simulink model "cbuildv3p1"  (R2024b)
settings: Solver=VariableStepAuto  StartTime=0.0  StopTime=2  RelTol=1e-3
model workspace (MAT data in the model file):
  A_busbar = 0.0015
  A_pack = 0.711626248
  C = 400
  C_nominal = 3
  GR = 13.75
  I_max = 157.708978328
  Izz = 76.97
  M = 251.54
  P = 5
  P_DD = 1
  REGEN_GAIN = 1
  R_e = 0.195
  S = 138
  SW_TV_GAIN = 0.0250298750679
  SoC_initial = 1
  TC_CUT = 500
  T_amb = 297.15
  Tmax = 21
  W = 1.53
  W_max = 34
  a = 0.7497
  busbar_CC_area = 0.000108
  busbar_Cp = 237
  busbar_length = 0.032
  busbar_mass = 0.01
  busbar_resistivity = 1.68e-08
  busbar_thermalcontact_resistance = 1
  c_factor = 0.244
  cell_Cp = 1000
  cell_mass = 0.046
  deg_to_rad = 0.0174533
  g = 9.81
  h = 0.253
  h_busbar = 5
  h_pack = 5
  kappa_thresh = 0.05
  l = 1.53
  mpersec_to_kph = 3.6
  rackdisp_to_steerangle = 1.29615626969
  rad_to_deg = 57.2958
  rpm_to_radpers = 0.10472
  t = 1.2
libraries: Solver_SF x1
(part 1 of 2)
settings Model: Creator=account  LastModifiedBy=kara.28

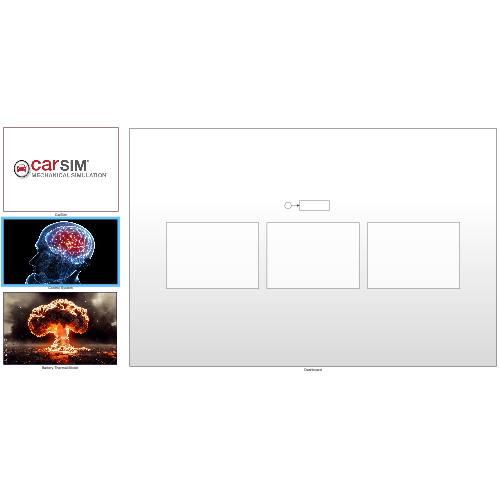
[thumbnail: Simulink's stored preview of the top-level diagram]
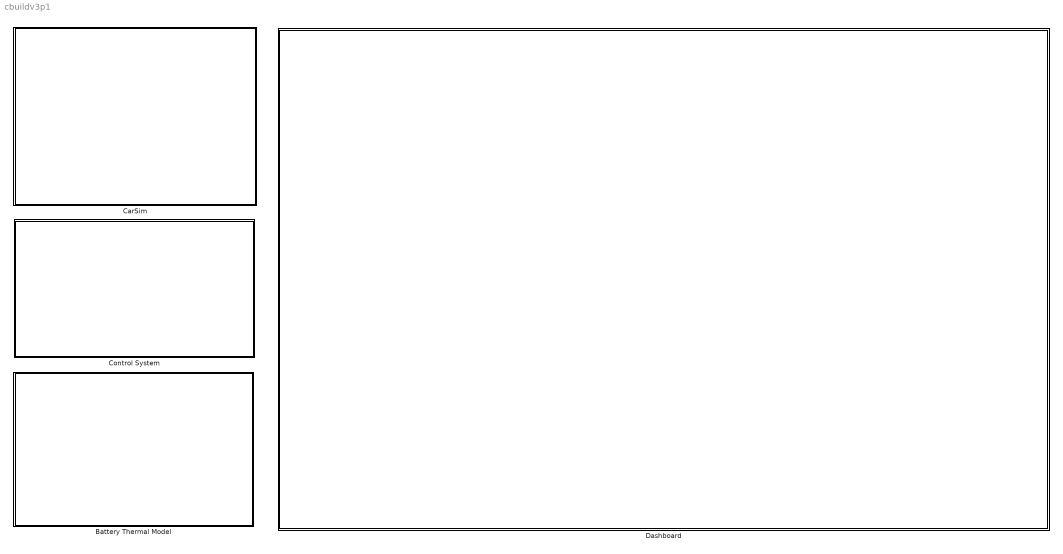
== system cbuildv3p1 ==
  Battery Thermal Model : Subsystem
      mask Display: image('battery.jpg');
  CarSim : Subsystem
      mask Display: image('carsimlogo.jpg');
  Control System : Subsystem
      mask Display: image('controller.jpg');
  Dashboard : Subsystem

== system cbuildv3p1/Battery Thermal Model ==
  Battery Cells : Subsystem
  Busbars : Subsystem

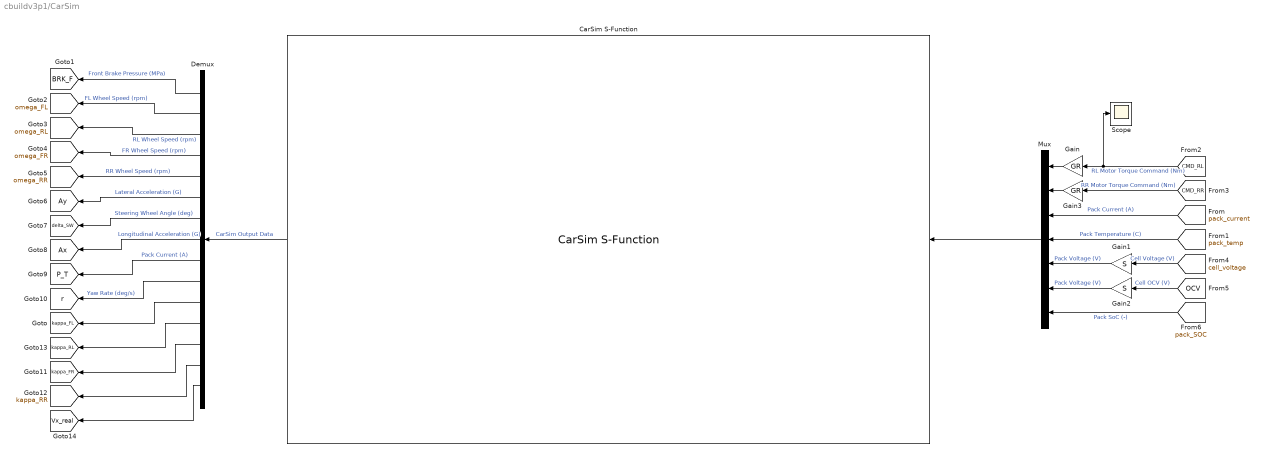
== system cbuildv3p1/CarSim ==
  CarSim S-Function : Solver_SF/CarSim S-Function  Priority=1  SIMFILE=simfile.sim  Run_RTs=off  vs_state_ind=Run  StopMode_ind=Vehicle Model
  Demux : Demux  Outputs=15
  Gain : Gain  Gain=GR
  Gain1 : Gain  Gain=S
  Gain2 : Gain  Gain=S
  Gain3 : Gain  Gain=GR
  Mux : Mux  Inputs=7
  Scope : Scope
  tag scope: Ax=global, Ay=global, BRK_F=global, P_T=global, Vx_real=global, delta_SW=global, kappa_FL=global, kappa_FR=global, kappa_RL=global, kappa_RR=global, omega_FL=global, omega_FR=global, omega_RL=global, omega_RR=global, r=global
  wires:
  Demux/5 -> [omega_RR]  "RR Wheel Speed (rpm)"
  Demux/8 -> [Ax]  "Longitudinal Acceleration (G)"
  Demux/4 -> [omega_FR]  "FR Wheel Speed (rpm)"
  Demux/2 -> [omega_FL]  "FL Wheel Speed (rpm)"
  CarSim S-Function/1 -> Demux/1  "CarSim Output Data"
  Demux/7 -> [delta_SW]  "Steering Wheel Angle (deg)"
  [CMD_RR] -> Gain3/1  "RR Motor Torque Command (Nm)"
  [CMD_RL] -> Scope/1, Gain/1  "RL Motor Torque Command (Nm)"
  Demux/3 -> [omega_RL]  "RL Wheel Speed (rpm)"
  Demux/1 -> [BRK_F]  "Front Brake Pressure (MPa)"
  Demux/6 -> [Ay]  "Lateral Acceleration (G)"
  Mux/1 -> CarSim S-Function/1
  Demux/10 -> [r]  "Yaw Rate (deg/s)"
  [pack_current] -> Mux/3  "Pack Current (A)"
  [pack_temp] -> Mux/4  "Pack Temperature (C)"
  [pack_SOC] -> Mux/7  "Pack SoC (-)"
  [OCV] -> Gain2/1  "Cell OCV (V)"
  [cell_voltage] -> Gain1/1  "Cell Voltage (V)"
  Gain1/1 -> Mux/5  "Pack Voltage (V)"
  Gain2/1 -> Mux/6  "Pack Voltage (V)"
  Gain/1 -> Mux/1
  Gain3/1 -> Mux/2
  Demux/9 -> [P_T]  "Pack Current (A)"
  Demux/11 -> [kappa_FL]
  Demux/12 -> [kappa_RL]
  Demux/13 -> [kappa_FR]
  Demux/14 -> [kappa_RR]
  Demux/15 -> [Vx_real]

== system cbuildv3p1/Control System ==
  Driver Assists : Subsystem
      settings: PortSchema="{\"entries\":[{\"content\":{\"sides\":[{\"content\":{\"connectorIds\":[\"In1\",\"In2\"]},\"type\":\"ConnectorPlacement.EquallySpacedRectSide\",\"uuid\":\"c30f5bbb-5f7b-4b8f-a220-579b9cc0865f\"},{\"content\":{\"connectorIds\":[\"Out1\",\"Out2\"],\"side\":\"RIGHT\"},\"type\":\"ConnectorPlacement.EquallySpacedRectSide\",\"uuid\":\"8399a92e-19c3-49c4-801c-f7e7f76799cf\"},{\"content\":{\"connectorIds\":[\"In3\",\"In4\",\"In5\",\"In6\",\"In7\",\"In8\",\"In9\"],\"side\":\"TOP\"},\"type\":\"ConnectorPlacement.EquallySpacedRectSide\",\"uuid\":\"19d8375b-8353-4f23-adee-fcd0b0fbd4ef\"}]},\"type\":\"ConnectorPlacement.EquallySpacedConnector\",\"uuid\":\"53834b5a-6686-42bc-a078-9cae71bfd001\"}],\"packageUris\":[\"http://schema.mathworks.com/mf0/Connector/R2020b\"],\"version\":\"1.0\"}"
  Dynamic Derate Dial Position : Constant
  Energy Management System : Subsystem
      settings: PortSchema="{\"entries\":[{\"content\":{\"sides\":[{\"content\":{\"connectorIds\":[\"In1\",\"In2\"]},\"type\":\"ConnectorPlacement.EquallySpacedRectSide\",\"uuid\":\"89c92abe-ca77-4c48-ba79-1fd8447b36ee\"},{\"content\":{\"connectorIds\":[\"Out1\",\"Out2\"],\"side\":\"RIGHT\"},\"type\":\"ConnectorPlacement.EquallySpacedRectSide\",\"uuid\":\"4a58accb-bbe3-490f-b1ea-5257f75ab2ba\"},{\"content\":{\"connectorIds\":[\"In3\",\"In4\",\"In5\"],\"side\":\"TOP\"},\"type\":\"ConnectorPlacement.EquallySpacedRectSide\",\"uuid\":\"b5e96e52-1098-4ccd-9740-b2b10d8cf6b3\"}]},\"type\":\"ConnectorPlacement.EquallySpacedConnector\",\"uuid\":\"06c6d35a-fc7b-4382-b862-8bbe65743431\"}],\"packageUris\":[\"http://schema.mathworks.com/mf0/Connector/R2020b\"],\"version\":\"1.0\"}"
  tag scope: CMD_RL=global, CMD_RR=global
  wires:
  Energy Management System/1(CMD_R) -> Driver Assists/1(CMD_R)
  Energy Management System/2(Tmax) -> Driver Assists/2(Tmax)
  Driver Assists/1(CMD_RL) -> [CMD_RL]
  Driver Assists/2(CMD_RR) -> [CMD_RR]
  [pack_temp] -> Energy Management System/1(T_BAT_MAX)  "Battery Temp (C)"
  Dynamic Derate Dial Position/1 -> Energy Management System/2(P_DD)  "Derate Dial Position (-)"
  [omega_RR] -> Driver Assists/6(omega_RR), Energy Management System/5(omega_RR)  "RR Wheel Speed (rpm)"
  [omega_FR] -> Driver Assists/4(omega_FR)  "FR Wheel Speed (rpm)"
  [omega_RL] -> Driver Assists/5(omega_RL), Energy Management System/3(omega_RL)  "RL Wheel Speed (rpm)"
  [omega_FL] -> Driver Assists/3(omega_FL)  "FL Wheel Speed (rpm)"
  [P_T] -> Driver Assists/7(P_T)  "Throttle Position (-)"
  [Ay] -> Driver Assists/8(Ax)  "Lateral Acceleration (G)"
  [BRK_F] -> Energy Management System/4(BRK_F), Driver Assists/9(BRK_F)  "Front Brake Pressure (MPa)"

== system cbuildv3p1/Dashboard ==
  Battery Info : Subsystem
  Clock1 : Clock
  Controls Info : Subsystem
  General Info : Subsystem
  Simulation Time : Display
  wires:
  Clock1/1 -> Simulation Time/1

== system cbuildv3p1/Battery Thermal Model/Battery Cells ==
  Battery Heat : Subsystem
      settings: PortSchema="{\"entries\":[{\"content\":{\"sides\":[{\"content\":{\"connectorIds\":[\"In1\",\"Out1\",\"In2\",\"In3\"]},\"type\":\"ConnectorPlacement.EquallySpacedRectSide\",\"uuid\":\"0f7c0562-63f7-413a-9c65-7d5d0f23ac53\"},{\"content\":{\"side\":\"RIGHT\"},\"type\":\"ConnectorPlacement.EquallySpacedRectSide\",\"uuid\":\"6856fc4a-e601-47fb-aafe-3183d6398fa2\"},{\"content\":{\"side\":\"TOP\"},\"type\":\"ConnectorPlacement.EquallySpacedRectSide\",\"uuid\":\"93500152-ab0c-4e86-a765-8796b82b9cd6\"}]},\"type\":\"ConnectorPlacement.EquallySpacedConnector\",\"uuid\":\"8bef09a8-0835-4033-ba4e-3f5f6277d0ac\"}],\"packageUris\":[\"http://schema.mathworks.com/mf0/Connector/R2020b\"],\"version\":\"1.0\"}"
  Battery Heat Generation : Subsystem
  Busbar - Segment Heat Flow : Subsystem
      settings: PortSchema="{\"entries\":[{\"content\":{\"sides\":[{\"content\":{},\"type\":\"ConnectorPlacement.EquallySpacedRectSide\",\"uuid\":\"839c7b7c-3d90-4543-803d-828e2cd8ee3e\"},{\"content\":{\"connectorIds\":[\"In1\",\"Out1\"],\"side\":\"RIGHT\"},\"type\":\"ConnectorPlacement.EquallySpacedRectSide\",\"uuid\":\"e3492608-3f40-473c-8392-0c925b682872\"},{\"content\":{\"side\":\"TOP\"},\"type\":\"ConnectorPlacement.EquallySpacedRectSide\",\"uuid\":\"8e15337c-e61d-491c-b508-620217c9bb60\"}]},\"type\":\"ConnectorPlacement.EquallySpacedConnector\",\"uuid\":\"03d3ec16-7a24-4203-9805-446eb586226e\"}],\"packageUris\":[\"http://schema.mathworks.com/mf0/Connector/R2020b\"],\"version\":\"1.0\"}"
  Heat Loss : Subsystem
      settings: PortSchema="{\"entries\":[{\"content\":{\"sides\":[{\"content\":{},\"type\":\"ConnectorPlacement.EquallySpacedRectSide\",\"uuid\":\"cd11f8f0-ebc0-4dda-8c98-00f5919de41a\"},{\"content\":{\"connectorIds\":[\"In1\",\"Out1\"],\"side\":\"RIGHT\"},\"type\":\"ConnectorPlacement.EquallySpacedRectSide\",\"uuid\":\"2a68a9a1-bd97-4a17-8a8b-1aa98e9bd9a8\"},{\"content\":{\"side\":\"TOP\"},\"type\":\"ConnectorPlacement.EquallySpacedRectSide\",\"uuid\":\"debcc510-941b-4448-a371-f67c84c59f32\"}]},\"type\":\"ConnectorPlacement.EquallySpacedConnector\",\"uuid\":\"91559e46-754b-48b4-ac3e-ab135f9add0a\"}],\"packageUris\":[\"http://schema.mathworks.com/mf0/Connector/R2020b\"],\"version\":\"1.0\"}"
  wires:
  Battery Heat/1(Pack Temp (K)) -> Busbar - Segment Heat Flow/1(Segment Temp (K)), Heat Loss/1(Pack Temp (K))
  Battery Heat Generation/1(Battery Heat Generation Rate) -> Battery Heat/1(Battery Heat Generation)
  Heat Loss/1(Pack Heat Loss Rate) -> Battery Heat/2(Battery Heat Loss)
  Busbar - Segment Heat Flow/1(Busbar - Segment Heat Flow (W)) -> Battery Heat/3(Busbar - Segment Heat Flow (W))

== system cbuildv3p1/Battery Thermal Model/Busbars ==
  Ambient Heat Loss : Subsystem
      settings: PortSchema="{\"entries\":[{\"content\":{\"sides\":[{\"content\":{},\"type\":\"ConnectorPlacement.EquallySpacedRectSide\",\"uuid\":\"cd11f8f0-ebc0-4dda-8c98-00f5919de41a\"},{\"content\":{\"connectorIds\":[\"In1\",\"Out1\"],\"side\":\"RIGHT\"},\"type\":\"ConnectorPlacement.EquallySpacedRectSide\",\"uuid\":\"2a68a9a1-bd97-4a17-8a8b-1aa98e9bd9a8\"},{\"content\":{\"side\":\"TOP\"},\"type\":\"ConnectorPlacement.EquallySpacedRectSide\",\"uuid\":\"debcc510-941b-4448-a371-f67c84c59f32\"}]},\"type\":\"ConnectorPlacement.EquallySpacedConnector\",\"uuid\":\"91559e46-754b-48b4-ac3e-ab135f9add0a\"}],\"packageUris\":[\"http://schema.mathworks.com/mf0/Connector/R2020b\"],\"version\":\"1.0\"}"
  Busbar - Segment Heat Flow : Subsystem
      settings: PortSchema="{\"entries\":[{\"content\":{\"sides\":[{\"content\":{},\"type\":\"ConnectorPlacement.EquallySpacedRectSide\",\"uuid\":\"839c7b7c-3d90-4543-803d-828e2cd8ee3e\"},{\"content\":{\"connectorIds\":[\"In1\",\"Out1\"],\"side\":\"RIGHT\"},\"type\":\"ConnectorPlacement.EquallySpacedRectSide\",\"uuid\":\"e3492608-3f40-473c-8392-0c925b682872\"},{\"content\":{\"side\":\"TOP\"},\"type\":\"ConnectorPlacement.EquallySpacedRectSide\",\"uuid\":\"8e15337c-e61d-491c-b508-620217c9bb60\"}]},\"type\":\"ConnectorPlacement.EquallySpacedConnector\",\"uuid\":\"03d3ec16-7a24-4203-9805-446eb586226e\"}],\"packageUris\":[\"http://schema.mathworks.com/mf0/Connector/R2020b\"],\"version\":\"1.0\"}"
  Busbar Heat : Subsystem
      settings: PortSchema="{\"entries\":[{\"content\":{\"sides\":[{\"content\":{\"connectorIds\":[\"In1\",\"Out1\",\"In2\",\"In3\"]},\"type\":\"ConnectorPlacement.EquallySpacedRectSide\",\"uuid\":\"0f7c0562-63f7-413a-9c65-7d5d0f23ac53\"},{\"content\":{\"side\":\"RIGHT\"},\"type\":\"ConnectorPlacement.EquallySpacedRectSide\",\"uuid\":\"6856fc4a-e601-47fb-aafe-3183d6398fa2\"},{\"content\":{\"side\":\"TOP\"},\"type\":\"ConnectorPlacement.EquallySpacedRectSide\",\"uuid\":\"93500152-ab0c-4e86-a765-8796b82b9cd6\"}]},\"type\":\"ConnectorPlacement.EquallySpacedConnector\",\"uuid\":\"8bef09a8-0835-4033-ba4e-3f5f6277d0ac\"}],\"packageUris\":[\"http://schema.mathworks.com/mf0/Connector/R2020b\"],\"version\":\"1.0\"}"
  Resistance Heat Generation : Subsystem
  wires:
  Busbar Heat/1(Busbar Temp (K)) -> Busbar - Segment Heat Flow/1(Busbar Temp (K)), Ambient Heat Loss/1(Busbar Temp (K))
  Resistance Heat Generation/1(Busbar Heat Generation Rate) -> Busbar Heat/1(Busbar Heat Generation)
  Ambient Heat Loss/1(Busbar Heat Loss Rate) -> Busbar Heat/2(Busbar Heat Loss)
  Busbar - Segment Heat Flow/1(Busbar - Segment Heat Flow (W)) -> Busbar Heat/3(Busbar - Segment Heat Flow (W))

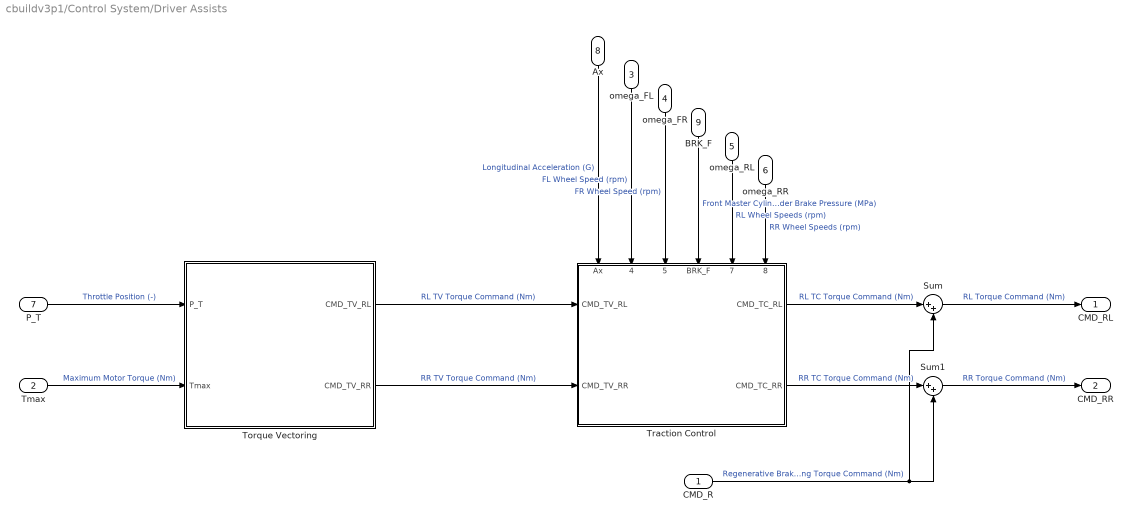
== system cbuildv3p1/Control System/Driver Assists ==
  CMD_R : Inport
  Tmax : Inport  Port=2
  omega_FL : Inport  Port=3
  omega_FR : Inport  Port=4
  omega_RL : Inport  Port=5
  omega_RR : Inport  Port=6
  P_T : Inport  Port=7
  Ax : Inport  Port=8
  BRK_F : Inport  Port=9
  Sum : Sum  Inputs=|++
  Sum1 : Sum  Inputs=|++
  Torque Vectoring : Subsystem
  Traction Control : Subsystem
      settings: PortSchema="{\"entries\":[{\"content\":{\"sides\":[{\"content\":{\"connectorIds\":[\"In1\",\"In2\"]},\"type\":\"ConnectorPlacement.EquallySpacedRectSide\",\"uuid\":\"d61c18bd-9535-4dda-869d-17effaf93de7\"},{\"content\":{\"connectorIds\":[\"Out1\",\"Out2\"],\"side\":\"RIGHT\"},\"type\":\"ConnectorPlacement.EquallySpacedRectSide\",\"uuid\":\"01ce504d-a060-4358-8411-664eedaba102\"},{\"content\":{\"connectorIds\":[\"In3\",\"In4\",\"In5\",\"In6\",\"In7\",\"In8\"],\"side\":\"TOP\"},\"type\":\"ConnectorPlacement.EquallySpacedRectSide\",\"uuid\":\"26eb6c05-86e8-47d0-a1b5-f53131bb5e60\"}]},\"type\":\"ConnectorPlacement.EquallySpacedConnector\",\"uuid\":\"a0cd41b8-03b3-4f62-a25e-73ac641935b2\"}],\"packageUris\":[\"http://schema.mathworks.com/mf0/Connector/R2020b\"],\"version\":\"1.0\"}"
  CMD_RL : Outport
  CMD_RR : Outport  Port=2
  wires:
  Torque Vectoring/2(CMD_TV_RR) -> Traction Control/2(CMD_TV_RR)  "RR TV Torque Command (Nm)"
  P_T/1 -> Torque Vectoring/1(P_T)  "Throttle Position (-)"
  Tmax/1 -> Torque Vectoring/2(Tmax)  "Maximum Motor Torque (Nm)"
  Sum/1 -> CMD_RL/1  "RL Torque Command (Nm)"
  Sum1/1 -> CMD_RR/1  "RR Torque Command (Nm)"
  CMD_R/1 -> Sum/2, Sum1/2  "Regenerative Braking Torque Command (Nm)"
  Ax/1 -> Traction Control/3(Ax)  "Longitudinal Acceleration (G)"
  omega_FL/1 -> Traction Control/4(omega_FL)  "FL Wheel Speed (rpm)"
  omega_FR/1 -> Traction Control/5(omega_FR)  "FR Wheel Speed (rpm)"
  BRK_F/1 -> Traction Control/6(BRK_F)  "Front Master Cylinder Brake Pressure (MPa)"
  omega_RL/1 -> Traction Control/7(omega_RL)  "RL Wheel Speeds (rpm)"
  omega_RR/1 -> Traction Control/8(omega_RR)  "RR Wheel Speeds (rpm)"
  Torque Vectoring/1(CMD_TV_RL) -> Traction Control/1(CMD_TV_RL)  "RL TV Torque Command (Nm)"
  Traction Control/1(CMD_TC_RL) -> Sum/1  "RL TC Torque Command (Nm)"
  Traction Control/2(CMD_TC_RR) -> Sum1/1  "RR TC Torque Command (Nm)"

== system cbuildv3p1/Control System/Energy Management System ==
  T_BAT_MAX : Inport
  P_DD : Inport  Port=2
  omega_RL : Inport  Port=3
  BRK_F : Inport  Port=4
  omega_RR : Inport  Port=5
  Dynamic Derate : Subsystem
  Regenerative Braking : Subsystem
  CMD_R : Outport
  Tmax : Outport  Port=2
  wires:
  T_BAT_MAX/1 -> Dynamic Derate/1(T_BAT_MAX)  "Maximum Module Temp (C)"
  P_DD/1 -> Dynamic Derate/2(P_DD)  "Dynamic Derate Dial Position (-)"
  BRK_F/1 -> Regenerative Braking/1(BRK_F)  "Front Master Cylinder Pressure (MPa)"
  Dynamic Derate/1(Tmax) -> Tmax/1  "Maximum Motor Torque (Nm)"
  Regenerative Braking/1(CMD_R) -> CMD_R/1  "Regen Brake Torque Command (Nm)"
  omega_RL/1 -> Dynamic Derate/3(omega_RL)  "RL Wheel Speed (rpm)"
  omega_RR/1 -> Dynamic Derate/4(omega_RR)  "RR Wheel Speed (rpm)"

== system cbuildv3p1/Dashboard/Battery Info ==
  Acceleration Scope : DashboardScope  Ymin=-2.5  Ymax=2.5
  Acceleration Scope1 : DashboardScope  Ymin=0  Ymax=60
  Acceleration Scope2 : DashboardScope  Ymin=0  Ymax=1
  Acceleration Scope3 : DashboardScope  Ymin=0  Ymax=1
  Acceleration Scope4 : DashboardScope  Ymin=0  Ymax=500

== system cbuildv3p1/Dashboard/Controls Info ==
  Acceleration Scope : DashboardScope  Ymin=-2.5  Ymax=2.5
  Acceleration Scope1 : DashboardScope  Ymin=-2  Ymax=2
  Acceleration Scope2 : DashboardScope  Ymin=0  Ymax=1
  Acceleration Scope3 : DashboardScope  Ymin=0  Ymax=80
  Acceleration Scope4 : DashboardScope  Ymin=0  Ymax=21
  Lamp : LampBlock  LabelPosition=Hide
  Rotary Switch : RotarySwitchBlock
      settings: Values={{'DD 1', 'DD 2'}, [0 1]}

== system cbuildv3p1/Dashboard/General Info ==
  Acceleration Scope : DashboardScope  Ymin=-2.5  Ymax=2.5
  Acceleration Scope1 : DashboardScope  Ymin=0  Ymax=110
  Acceleration Scope2 : DashboardScope  Ymin=0  Ymax=1
  Acceleration Scope3 : DashboardScope  Ymin=0  Ymax=10

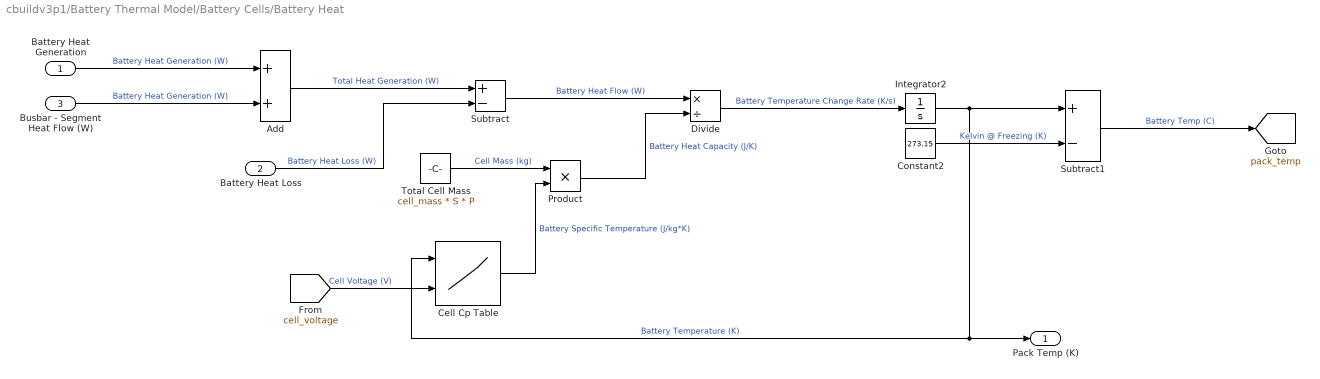
== system cbuildv3p1/Battery Thermal Model/Battery Cells/Battery Heat ==
  Battery Heat Generation : Inport
  Battery Heat Loss : Inport  Port=2
  Busbar - Segment Heat Flow (W) : Inport  Port=3
  Add : Sum
  Cell Cp Table : Lookup_n-D  BreakpointsForDimension1=[296.0488;303.3425;312.147;321.5769;330.6423]  BreakpointsForDimension2=[0 0.5 1]  Table=[811.0868 819.6535 830.8545;814.1373 822.704 834.6964;817.9826 826.8129 838.6737000000001;822.2249 831.0552 843.4446;826.7299 835.8239 848.3459]  InterpMethod=Cubic spline  InternalRulePriority=Speed  RndMeth=Simplest
      settings: InputPortMap=u0,u1
  Constant2 : Constant  Value=273.15
  Divide : Product  Inputs=*/
  Integrator2 : Integrator  InitialCondition=T_amb
  Product : Product
  Subtract : Sum  Inputs=+-
  Subtract1 : Sum  Inputs=+-
  Total Cell Mass : Constant  Value=cell_mass * S * P
  Pack Temp (K) : Outport
  tag scope: pack_temp=global
  wires:
  Cell Cp Table/1 -> Product/2  "Battery Specific Temperature (J/kg*K)"
  Constant2/1 -> Subtract1/2  "Kelvin @ Freezing (K)"
  Divide/1 -> Integrator2/1  "Battery Temperature Change Rate (K/s)"
  Subtract/1 -> Divide/1  "Battery Heat Flow (W)"
  Integrator2/1 -> Cell Cp Table/1, Pack Temp (K)/1, Subtract1/1  "Battery Temperature (K)"
  Subtract1/1 -> [pack_temp]  "Battery Temp (C)"
  Total Cell Mass/1 -> Product/1  "Cell Mass (kg)"
  Product/1 -> Divide/2  "Battery Heat Capacity (J/K)"
  Battery Heat Loss/1 -> Subtract/2  "Battery Heat Loss (W)"
  Battery Heat Generation/1 -> Add/1  "Battery Heat Generation (W)"
  Busbar - Segment Heat Flow (W)/1 -> Add/2  "Battery Heat Generation (W)"
  Add/1 -> Subtract/1  "Total Heat Generation (W)"
  [cell_voltage] -> Cell Cp Table/2  "Cell Voltage (V)"

== system cbuildv3p1/Battery Thermal Model/Battery Cells/Battery Heat Generation ==
  Cell Resistance : Subsystem
      settings: PortSchema="{\"entries\":[{\"content\":{\"sides\":[{\"content\":{},\"type\":\"ConnectorPlacement.EquallySpacedRectSide\",\"uuid\":\"1c6ff2a8-2c86-4b92-aa7d-5717a02d6f28\"},{\"content\":{\"connectorIds\":[\"In1\",\"In2\",\"Out1\"],\"side\":\"RIGHT\"},\"type\":\"ConnectorPlacement.EquallySpacedRectSide\",\"uuid\":\"52a4cb2c-e1db-459d-bd0a-206cc3bba6d1\"},{\"content\":{\"side\":\"TOP\"},\"type\":\"ConnectorPlacement.EquallySpacedRectSide\",\"uuid\":\"751bbbd6-abc7-4265-8d68-4aa70d69379f\"}]},\"type\":\"ConnectorPlacement.EquallySpacedConnector\",\"uuid\":\"b8f9630f-0167-4478-8d98-637e13782dcd\"}],\"packageUris\":[\"http://schema.mathworks.com/mf0/Connector/R2020b\"],\"version\":\"1.0\"}"
      mask Display: image('resistor.png');
  Cells in Parallel : Constant  Value=P
  Cells in series : Constant  Value=S
  Divide : Product  Inputs=*/
  Pack Current : Subsystem
      mask Display: image('current.png');
  Pack SoC : Subsystem
      settings: PortSchema="{\"entries\":[{\"content\":{\"sides\":[{\"content\":{},\"type\":\"ConnectorPlacement.EquallySpacedRectSide\",\"uuid\":\"1c6ff2a8-2c86-4b92-aa7d-5717a02d6f28\"},{\"content\":{\"connectorIds\":[\"In1\",\"Out1\"],\"side\":\"RIGHT\"},\"type\":\"ConnectorPlacement.EquallySpacedRectSide\",\"uuid\":\"52a4cb2c-e1db-459d-bd0a-206cc3bba6d1\"},{\"content\":{\"side\":\"TOP\"},\"type\":\"ConnectorPlacement.EquallySpacedRectSide\",\"uuid\":\"751bbbd6-abc7-4265-8d68-4aa70d69379f\"}]},\"type\":\"ConnectorPlacement.EquallySpacedConnector\",\"uuid\":\"b8f9630f-0167-4478-8d98-637e13782dcd\"}],\"packageUris\":[\"http://schema.mathworks.com/mf0/Connector/R2020b\"],\"version\":\"1.0\"}"
      mask Display: image('SoC.jpg');
  Product : Product
  Product1 : Product
  Product2 : Product
  Square : Math  Operator=square
  Battery Heat Generation Rate : Outport
  wires:
  Cells in series/1 -> Product1/1
  Divide/1 -> Cell Resistance/1(Cell Current  (A)), Square/1  "Cell Current (A)"
  Cell Resistance/1(Cell Resistance (ohms)) -> Product/2  "Cell Resistance (ohms)"
  Square/1 -> Product/1
  Cells in Parallel/1 -> Divide/2, Product1/2
  Product1/1 -> Product2/2
  Product/1 -> Product2/1  "Cell Heat Generation Rate (W)"
  Product2/1 -> Battery Heat Generation Rate/1  "Pack Heat Generation Rate (W)"
  Pack SoC/1(SoC (%)) -> Cell Resistance/2(SoC (%))  "Pack SoC (%)"
  Pack Current/1(Pack Current (A)) -> Divide/1, Pack SoC/1(Pack Current (A))  "Pack Current (A)"

== system cbuildv3p1/Battery Thermal Model/Battery Cells/Busbar - Segment Heat Flow ==
  Segment Temp (K) : Inport
  Add : Sum
  Kelvin @ 0C : Constant  Value=273.15
  Product : Product
  Subtract : Sum  Inputs=+-
  Thermal Capacitance  (W/K) : Constant  Value=busbar_thermalcontact_resistance
  Busbar - Segment Heat Flow (W) : Outport
  wires:
  Subtract/1 -> Product/1  "Temperature difference (K)"
  Thermal Capacitance  (W/K)/1 -> Product/2  "Thermal Capacitance (W/K)"
  Product/1 -> Busbar - Segment Heat Flow (W)/1  "Busbar - Segment Heat Flow (W)"
  [busbar_temp] -> Add/2  "Segment temp (C)"
  Kelvin @ 0C/1 -> Add/1  "Kelvin at Freezing (K)"
  Segment Temp (K)/1 -> Subtract/1
  Add/1 -> Subtract/2  "Segment temp (K)"

== system cbuildv3p1/Battery Thermal Model/Battery Cells/Heat Loss ==
  Pack Temp (K) : Inport
  Ambient Temp (K) : Constant  Value=T_amb
  Pack Convective Heat Transfer Coefficient (W/m^2*K) : Constant  Value=h_pack
  Pack Surface Area (m^2) : Gain  Gain=A_pack
  Product : Product
  Subtract : Sum  Inputs=+-
  Pack Heat Loss Rate : Outport
  tag scope: pack_heatloss=global
  wires:
  Pack Convective Heat Transfer Coefficient (W/m^2*K)/1 -> Pack Surface Area (m^2)/1  "Pack Convective Heat Transfer Coefficient (W/m^2*K)"
  Subtract/1 -> Product/2  "Temperature Difference (K)"
  Pack Surface Area (m^2)/1 -> Product/1  "Heat Transfer Capacitance (W/K)"
  Product/1 -> [pack_heatloss], Pack Heat Loss Rate/1  "Pack Heat Loss Rate (W)"
  Pack Temp (K)/1 -> Subtract/1  "Pack Temp (K)"
  Ambient Temp (K)/1 -> Subtract/2  "Ambient Temp (K)"

== system cbuildv3p1/Battery Thermal Model/Busbars/Ambient Heat Loss ==
  Busbar Temp (K) : Inport
  Ambient temp (K) : Constant  Value=T_amb
  H busbar : Constant  Value=h_busbar
  Product : Product
  Subtract : Sum  Inputs=+-
  busbar area : Gain  Gain=A_busbar
  Busbar Heat Loss Rate : Outport
  tag scope: busbar_heatloss=global
  wires:
  H busbar/1 -> busbar area/1
  Subtract/1 -> Product/2
  busbar area/1 -> Product/1
  Product/1 -> [busbar_heatloss], Busbar Heat Loss Rate/1
  Busbar Temp (K)/1 -> Subtract/1
  Ambient temp (K)/1 -> Subtract/2

== system cbuildv3p1/Battery Thermal Model/Busbars/Busbar - Segment Heat Flow ==
  Busbar Temp (K) : Inport
  Add : Sum
  Constant : Constant  Value=busbar_thermalcontact_resistance
  Constant1 : Constant  Value=273.15
  Divide : Product  Inputs=*/
  Subtract : Sum  Inputs=+-
  Busbar - Segment Heat Flow (W) : Outport
  tag scope: busbar_segment_heatflow=global
  wires:
  Busbar Temp (K)/1 -> Subtract/2
  Subtract/1 -> Divide/1  "Temp diff (K)"
  Constant/1 -> Divide/2
  Divide/1 -> [busbar_segment_heatflow], Busbar - Segment Heat Flow (W)/1
  [pack_temp] -> Add/2  "Segment temp (C)"
  Constant1/1 -> Add/1
  Add/1 -> Subtract/1  "Segment temp (K)"

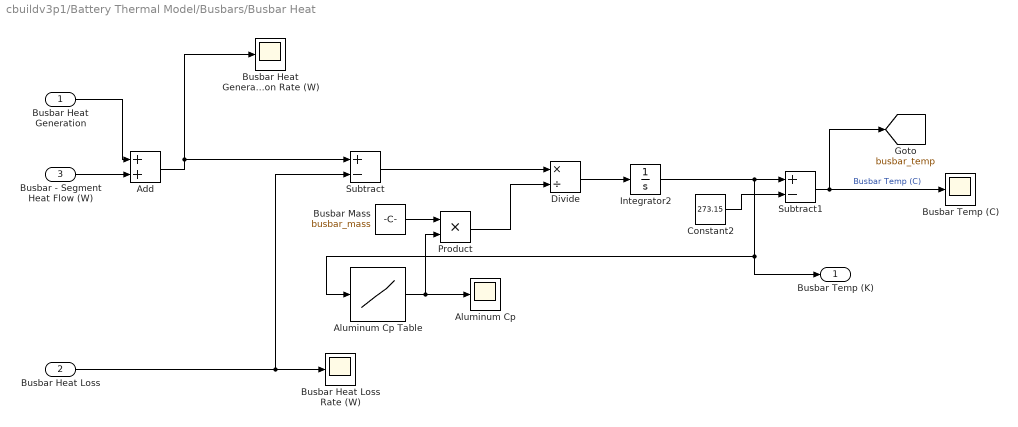
== system cbuildv3p1/Battery Thermal Model/Busbars/Busbar Heat ==
  Busbar Heat Generation : Inport
  Busbar Heat Loss : Inport  Port=2
  Busbar - Segment Heat Flow (W) : Inport  Port=3
  Add : Sum
  Aluminum Cp : Scope
  Aluminum Cp Table : Lookup_n-D  NumberOfTableDimensions=1  BreakpointsForDimension1=[298;300;400;500;600;700;800;900]  Table=[380.7;381.6;405.6;422.3;438.8;457.9;480.9;508.3]  InterpMethod=Cubic spline  InternalRulePriority=Speed  RndMeth=Simplest
  Busbar Heat Generation Rate (W) : Scope
  Busbar Heat Loss Rate (W) : Scope
  Busbar Mass : Constant  Value=busbar_mass
  Busbar Temp (C) : Scope
  Constant2 : Constant  Value=273.15
  Divide : Product  Inputs=*/
  Integrator2 : Integrator  InitialCondition=T_amb
  Product : Product
  Subtract : Sum  Inputs=+-
  Subtract1 : Sum  Inputs=+-
  Busbar Temp (K) : Outport
  tag scope: busbar_temp=global
  wires:
  Aluminum Cp Table/1 -> Product/2, Aluminum Cp/1
  Constant2/1 -> Subtract1/2
  Busbar Heat Generation/1 -> Add/1
  Divide/1 -> Integrator2/1
  Subtract/1 -> Divide/1
  Integrator2/1 -> Aluminum Cp Table/1, Busbar Temp (K)/1, Subtract1/1
  Subtract1/1 -> [busbar_temp], Busbar Temp (C)/1  "Busbar Temp (C)"
  Busbar Mass/1 -> Product/1
  Product/1 -> Divide/2
  Busbar Heat Loss/1 -> Busbar Heat Loss Rate (W)/1, Subtract/2
  Busbar - Segment Heat Flow (W)/1 -> Add/2
  Add/1 -> Subtract/1, Busbar Heat Generation Rate (W)/1

== system cbuildv3p1/Battery Thermal Model/Busbars/Resistance Heat Generation ==
  Busbar cross sectional area (m^2) : Constant  Value=busbar_CC_area
  Busbar length (m) : Constant  Value=busbar_length
  Busbar resistivity (Ohms * m) : Constant  Value=busbar_resistivity
  Divide : Product  Inputs=*/
  Product : Product
  Product1 : Product
  Square : Math  Operator=square
  Busbar Heat Generation Rate : Outport
  wires:
  Product/1 -> Busbar Heat Generation Rate/1  "Busbar Heat Loss (W)"
  [pack_current] -> Square/1  "Pack Current (A)"
  Square/1 -> Product/1
  Busbar resistivity (Ohms * m)/1 -> Product1/1
  Busbar length (m)/1 -> Product1/2
  Product1/1 -> Divide/1
  Busbar cross sectional area (m^2)/1 -> Divide/2
  Divide/1 -> Product/2  "Busbar resistance (ohms)"

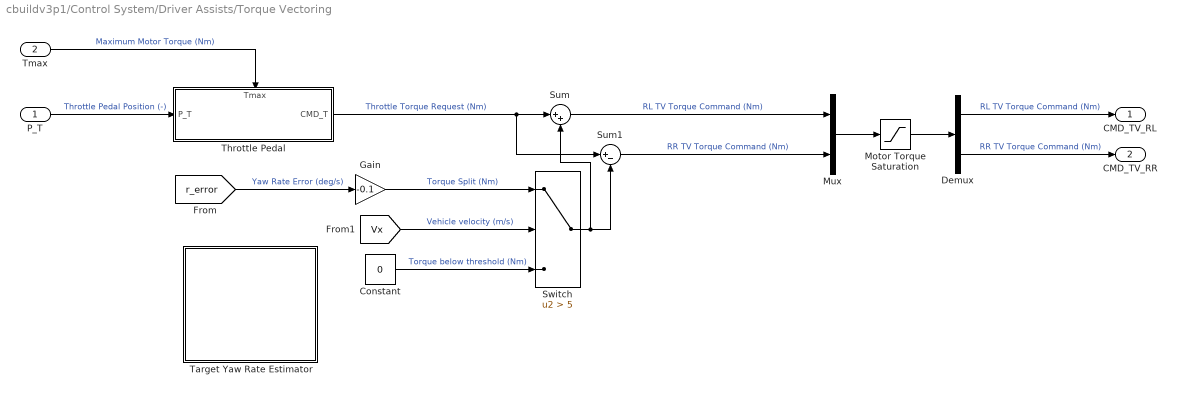
== system cbuildv3p1/Control System/Driver Assists/Torque Vectoring ==
  P_T : Inport
  Tmax : Inport  Port=2
  Constant : Constant  Value=0
  Demux : Demux  Outputs=2
  Gain : Gain  Gain=-0.1
  Motor Torque Saturation : Saturate  UpperLimit=Tmax  LowerLimit=-Tmax
  Mux : Mux  Inputs=2
  Sum : Sum  Inputs=|++
  Sum1 : Sum  Inputs=|+-
  Switch : Switch  Criteria=u2 > Threshold  Threshold=5  SaturateOnIntegerOverflow=off  InputSameDT=off
  Target Yaw Rate Estimator : Subsystem
  Throttle Pedal : Subsystem
      settings: PortSchema="{\"entries\":[{\"content\":{\"sides\":[{\"content\":{\"connectorIds\":[\"In1\"]},\"type\":\"ConnectorPlacement.EquallySpacedRectSide\",\"uuid\":\"2b27b7ae-a1b0-424c-ba89-4fa8e2fb9573\"},{\"content\":{\"connectorIds\":[\"Out1\"],\"side\":\"RIGHT\"},\"type\":\"ConnectorPlacement.EquallySpacedRectSide\",\"uuid\":\"35debb5b-e82d-4475-8dc9-1b915a5a0cae\"},{\"content\":{\"connectorIds\":[\"In2\"],\"side\":\"TOP\"},\"type\":\"ConnectorPlacement.EquallySpacedRectSide\",\"uuid\":\"f3fd2101-c365-4f42-b396-02e014a928b2\"}]},\"type\":\"ConnectorPlacement.EquallySpacedConnector\",\"uuid\":\"f19feaaa-e3f7-4392-8847-f37ac3c71c65\"}],\"packageUris\":[\"http://schema.mathworks.com/mf0/Connector/R2020b\"],\"version\":\"1.0\"}"
  CMD_TV_RL : Outport
  CMD_TV_RR : Outport  Port=2
  wires:
  Throttle Pedal/1(CMD_T) -> Sum1/1, Sum/1  "Throttle Torque Request (Nm)"
  Switch/1 -> Sum1/2, Sum/2
  Demux/1 -> CMD_TV_RL/1  "RL TV Torque Command (Nm)"
  Constant/1 -> Switch/3  "Torque below threshold (Nm)"
  Mux/1 -> Motor Torque Saturation/1
  Sum/1 -> Mux/1  "RL TV Torque Command (Nm)"
  P_T/1 -> Throttle Pedal/1(P_T)  "Throttle Pedal Position (-)"
  [r_error] -> Gain/1  "Yaw Rate Error (deg/s)"
  Motor Torque Saturation/1 -> Demux/1
  [Vx] -> Switch/2  "Vehicle velocity (m/s)"
  Tmax/1 -> Throttle Pedal/2(Tmax)  "Maximum Motor Torque (Nm)"
  Sum1/1 -> Mux/2  "RR TV Torque Command (Nm)"
  Gain/1 -> Switch/1  "Torque Split (Nm)"
  Demux/2 -> CMD_TV_RR/1  "RR TV Torque Command (Nm)"

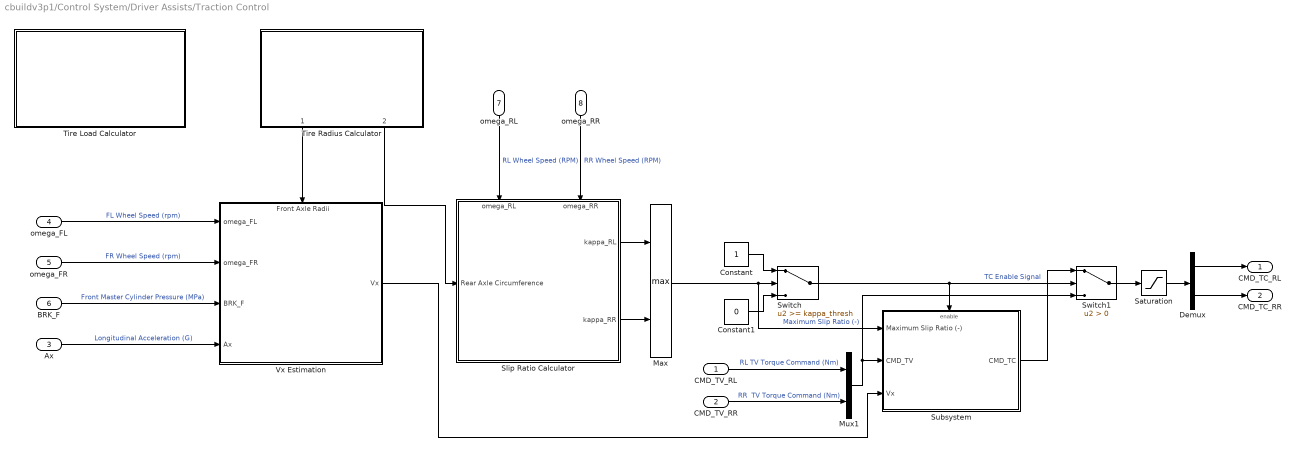
== system cbuildv3p1/Control System/Driver Assists/Traction Control ==
  CMD_TV_RL : Inport
  CMD_TV_RR : Inport  Port=2
  Ax : Inport  Port=3
  omega_FL : Inport  Port=4
  omega_FR : Inport  Port=5
  BRK_F : Inport  Port=6
  omega_RL : Inport  Port=7
  omega_RR : Inport  Port=8
  Constant : Constant
  Constant1 : Constant  Value=0
  Demux : Demux  Outputs=2
  Max : MinMax  Function=max  Inputs=2
  Mux1 : Mux  Inputs=2
  Saturation : Saturate  UpperLimit=Tmax  LowerLimit=-Tmax
  Slip Ratio Calculator : Subsystem
      settings: PortSchema="{\"entries\":[{\"content\":{\"sides\":[{\"content\":{\"connectorIds\":[\"In1\"]},\"type\":\"ConnectorPlacement.EquallySpacedRectSide\",\"uuid\":\"7fdfdad2-33dd-4f06-b604-3c6d01a9d7f8\"},{\"content\":{\"connectorIds\":[\"Out1\",\"Out2\"],\"side\":\"RIGHT\"},\"type\":\"ConnectorPlacement.EquallySpacedRectSide\",\"uuid\":\"dd7c3b4e-ee50-4427-819e-6ce97aa41bd4\"},{\"content\":{\"connectorIds\":[\"In2\",\"In3\"],\"side\":\"TOP\"},\"type\":\"ConnectorPlacement.EquallySpacedRectSide\",\"uuid\":\"78cf20ba-e7fd-4300-9f66-06aa85c1fb42\"}]},\"type\":\"ConnectorPlacement.EquallySpacedConnector\",\"uuid\":\"f81e5908-a010-4627-83b7-5417b93ce453\"}],\"packageUris\":[\"http://schema.mathworks.com/mf0/Connector/R2020b\"],\"version\":\"1.0\"}"
  Subsystem : Subsystem
  Switch : Switch  Threshold=kappa_thresh  SaturateOnIntegerOverflow=off  InputSameDT=off
  Switch1 : Switch  Criteria=u2 > Threshold  SaturateOnIntegerOverflow=off  InputSameDT=off
  Tire Load Calculator : Subsystem
  Tire Radius Calculator : Subsystem
      settings: PortSchema="{\"entries\":[{\"content\":{\"sides\":[{\"content\":{},\"type\":\"ConnectorPlacement.EquallySpacedRectSide\",\"uuid\":\"fb3f4c67-f54c-4634-ba2d-387163a9f315\"},{\"content\":{\"side\":\"RIGHT\"},\"type\":\"ConnectorPlacement.EquallySpacedRectSide\",\"uuid\":\"aebac900-8c66-4df6-bc19-49639b103298\"},{\"content\":{\"side\":\"TOP\"},\"type\":\"ConnectorPlacement.EquallySpacedRectSide\",\"uuid\":\"62c460bb-53fa-4252-8c13-d4e682a4bd0f\"},{\"content\":{\"connectorIds\":[\"Out1\",\"Out2\"],\"side\":\"BOTTOM\"},\"type\":\"ConnectorPlacement.EquallySpacedRectSide\",\"uuid\":\"783325cb-2928-4cef-a318-c835c1a005cf\"}]},\"type\":\"ConnectorPlacement.EquallySpacedConnector\",\"uuid\":\"2844ae35-273c-4d05-aae8-a401eaebcede\"}],\"packageUris\":[\"http://schema.mathworks.com/mf0/Connector/R2020b\"],\"version\":\"1.0\"}"
  Vx Estimation : Subsystem
      settings: PortSchema="{\"entries\":[{\"content\":{\"sides\":[{\"content\":{\"connectorIds\":[\"In1\",\"In2\",\"In3\",\"In4\"]},\"type\":\"ConnectorPlacement.EquallySpacedRectSide\",\"uuid\":\"62c79b25-0b9e-432c-bd58-3f819ebc25c7\"},{\"content\":{\"connectorIds\":[\"Out1\"],\"side\":\"RIGHT\"},\"type\":\"ConnectorPlacement.EquallySpacedRectSide\",\"uuid\":\"fa527cf3-b94d-4be1-9a9d-04b034fbf641\"},{\"content\":{\"connectorIds\":[\"In5\"],\"side\":\"TOP\"},\"type\":\"ConnectorPlacement.EquallySpacedRectSide\",\"uuid\":\"a12a099b-dd90-47cf-b0e3-d9aaf4967d5c\"}]},\"type\":\"ConnectorPlacement.EquallySpacedConnector\",\"uuid\":\"1196224d-9c5e-4514-ac5e-213e9ecc2f15\"}],\"packageUris\":[\"http://schema.mathworks.com/mf0/Connector/R2020b\"],\"version\":\"1.0\"}"
  CMD_TC_RL : Outport
  CMD_TC_RR : Outport  Port=2
  wires:
  Ax/1 -> Vx Estimation/4(Ax)  "Longitudinal Acceleration (G)"
  omega_FL/1 -> Vx Estimation/1(omega_FL)  "FL Wheel Speed (rpm)"
  omega_FR/1 -> Vx Estimation/2(omega_FR)  "FR Wheel Speed (rpm)"
  BRK_F/1 -> Vx Estimation/3(BRK_F)  "Front Master Cylinder Pressure (MPa)"
  omega_RL/1 -> Slip Ratio Calculator/2(omega_RL)  "RL Wheel Speed (RPM)"
  omega_RR/1 -> Slip Ratio Calculator/3(omega_RR)  "RR Wheel Speed (RPM)"
  Vx Estimation/1(Vx) -> Subsystem/3(Vx)
  Constant/1 -> Switch/1
  Constant1/1 -> Switch/3
  Switch/1 -> Switch1/2, Subsystem/Enable  "TC Enable Signal"
  Subsystem/1(CMD_TC) -> Switch1/1
  CMD_TV_RL/1 -> Mux1/1  "RL TV Torque Command (Nm)"
  CMD_TV_RR/1 -> Mux1/2  "RR  TV Torque Command (Nm)"
  Mux1/1 -> Switch1/3, Subsystem/2(CMD_TV)
  Switch1/1 -> Saturation/1
  Demux/1 -> CMD_TC_RL/1
  Demux/2 -> CMD_TC_RR/1
  Max/1 -> Subsystem/1(Maximum Slip Ratio (-)), Switch/2  "Maximum Slip Ratio (-)"
  Saturation/1 -> Demux/1
  Slip Ratio Calculator/2(kappa_RR) -> Max/2
  Slip Ratio Calculator/1(kappa_RL) -> Max/1
  Tire Radius Calculator/1(Front Axle Circumference) -> Vx Estimation/5("Front Axle Radii ")
  Tire Radius Calculator/2(Rear Axle Circumference) -> Slip Ratio Calculator/1(Rear Axle Circumference)

== system cbuildv3p1/Control System/Energy Management System/Dynamic Derate ==
  T_BAT_MAX : Inport
  P_DD : Inport  Port=2
  omega_RL : Inport  Port=3
  omega_RR : Inport  Port=4
  Dynamic Derate 3D LUT : Lookup_n-D  NumberOfTableDimensions=3  BreakpointsForDimension1=[0;25;50;75;100]  BreakpointsForDimension2=[30;50;60;80]  BreakpointsForDimension3=[1 2 3 4]  Table=reshape([80 80 80 80 80 80 80 80 80 80 80 80 80 80 80 80 80 80 80 80 73.5 73.5 73.5 73.5 73.5 60 60 50 40 30 40 40 30 20 15 20 15 12.5 10 10 36.75 36.75 36.75 36.75 36.75 30 30 25 20 15 20 20 15 10 7.5 10 7.5 6.25 5 5 18.375 18.375 18.375 18.375 18.375 15 15 12.5 10 7.5 10 10 7.5 5 3.75 5 3.75 3.125 2.5 2.5], [5 4 4])  ExtrapMethod=Clip  InternalRulePriority=Speed  RndMeth=Simplest
      settings: InputPortMap=u0,u1,u2
  Gain : Gain  Gain=mpersec_to_kph
  Motor Output Saturation : Saturate  UpperLimit=Tmax  LowerLimit=0
  Motor Torque Calculator : Subsystem
      settings: PortSchema="{\"entries\":[{\"content\":{\"sides\":[{\"content\":{\"connectorIds\":[\"In1\",\"In2\"]},\"type\":\"ConnectorPlacement.EquallySpacedRectSide\",\"uuid\":\"904eb794-76c4-4372-ae2c-4ef2e0000433\"},{\"content\":{\"connectorIds\":[\"Out1\"],\"side\":\"RIGHT\"},\"type\":\"ConnectorPlacement.EquallySpacedRectSide\",\"uuid\":\"8161fba4-68b1-4b44-95f9-b05533d0f86a\"},{\"content\":{\"connectorIds\":[\"In3\"],\"side\":\"TOP\"},\"type\":\"ConnectorPlacement.EquallySpacedRectSide\",\"uuid\":\"e37aa600-3bd6-4b73-8bba-520f94d37a3f\"}]},\"type\":\"ConnectorPlacement.EquallySpacedConnector\",\"uuid\":\"d8616461-ce1c-4b50-a881-919f614525dd\"}],\"packageUris\":[\"http://schema.mathworks.com/mf0/Connector/R2020b\"],\"version\":\"1.0\"}"
  Tmax : Outport
  wires:
  T_BAT_MAX/1 -> Dynamic Derate 3D LUT/1  "Maximum Module Temp (C)"
  [Vx] -> Gain/1
  P_DD/1 -> Dynamic Derate 3D LUT/3  "Dynamic Derate Dial Position (-)"
  Dynamic Derate 3D LUT/1 -> Motor Torque Calculator/3(B_MAX)  "Maximum Battery Power (KW)"
  omega_RL/1 -> Motor Torque Calculator/1(omega_RL)  "RL Wheel Speed (rpm)"
  omega_RR/1 -> Motor Torque Calculator/2(omega_RR)  "RR Wheel Speed (rpm)"
  Motor Torque Calculator/1(Tmax) -> Motor Output Saturation/1  "Maximum Motor Output Torque (Nm)"
  Motor Output Saturation/1 -> Tmax/1
  Gain/1 -> Dynamic Derate 3D LUT/2  "Vehicle Velocity (kph)"

== system cbuildv3p1/Control System/Energy Management System/Regenerative Braking ==
  BRK_F : Inport
  Regen Brake Torque Gain : Gain  Gain=REGEN_GAIN
  CMD_R : Outport
  wires:
  BRK_F/1 -> Regen Brake Torque Gain/1  "Front Master Cylinder Pressure (MPa)"
  Regen Brake Torque Gain/1 -> CMD_R/1  "Regen Brake Torque Command (Nm)"

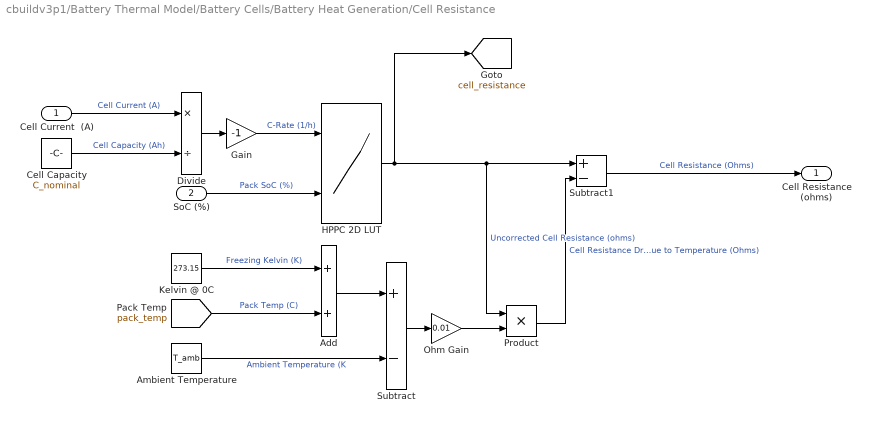
== system cbuildv3p1/Battery Thermal Model/Battery Cells/Battery Heat Generation/Cell Resistance ==
  Cell Current  (A) : Inport
  SoC (%) : Inport  Port=2
  Add : Sum
  Ambient Temperature : Constant  Value=T_amb
  Cell Capacity : Constant  Value=C_nominal
  Divide : Product  Inputs=*/
  Gain : Gain  Gain=-1
  HPPC 2D LUT : Lookup_n-D  BreakpointsForDimension1=[-10;-5;-1;1;2;3]  BreakpointsForDimension2=[0.1;0.2;0.3;0.4;0.5;0.6;0.7;0.8;0.9;1]  Table=[0.018906 0.01868 0.018453 0.018226 0.017999 0.017916 0.017743 0.018183 0.019549 0.022703;0.021356 0.020344 0.019332 0.019017 0.018694 0.018598 0.018319 0.018773 0.020642 0.024917;0.02305 0.020909 0.018859 0.019644 0.019687 0.018989 0.018291 0.019295 0.021608 0.026536;0.023001 0.020599 0.019683 0.019161 0.01894 0.018506 0.018636 0.019336 0.020993 0.02265;0.022654 0.020712 0.018901 0.018682 0.018442 0.018289 0.017788 0.017286 0.016785 0.016283;0.019898 0.017891 0.017366 0.01725 0.01725 0.017251 0.017251 0.017251 0.017251 0.017251]  InterpMethod=Cubic spline  ExtrapMethod=Clip  InternalRulePriority=Speed  RndMeth=Simplest
      settings: InputPortMap=u0,u1
  Kelvin @ 0C : Constant  Value=273.15
  Ohm Gain : Gain  Gain=0.01
  Product : Product
  Subtract : Sum  Inputs=+-
  Subtract1 : Sum  Inputs=+-
  Cell Resistance (ohms) : Outport
  tag scope: cell_resistance=global
  wires:
  Cell Current  (A)/1 -> Divide/1  "Cell Current (A)"
  Cell Capacity/1 -> Divide/2  "Cell Capacity (Ah)"
  SoC (%)/1 -> HPPC 2D LUT/2  "Pack SoC (%)"
  HPPC 2D LUT/1 -> [cell_resistance], Subtract1/1, Product/1  "Uncorrected Cell Resistance (ohms)"
  Divide/1 -> Gain/1
  Gain/1 -> HPPC 2D LUT/1  "C-Rate (1/h)"
  Subtract/1 -> Ohm Gain/1
  Ambient Temperature/1 -> Subtract/2  "Ambient Temperature (K"
  [pack_temp] -> Add/2  "Pack Temp (C)"
  Add/1 -> Subtract/1
  Kelvin @ 0C/1 -> Add/1  "Freezing Kelvin (K)"
  Ohm Gain/1 -> Product/2
  Product/1 -> Subtract1/2  "Cell Resistance Drop Due to Temperature (Ohms)"
  Subtract1/1 -> Cell Resistance (ohms)/1  "Cell Resistance (Ohms)"

== system cbuildv3p1/Battery Thermal Model/Battery Cells/Battery Heat Generation/Pack Current ==
  Divide : Product  Inputs=*/
  Gain : Gain  Gain=S
  Power Estimator : Subsystem
  Sony VTC6 Equivalent Circuit : Subsystem
  Pack Current (A) : Outport
  tag scope: pack_current=global
  wires:
  Power Estimator/1(Motor Power (W)) -> Divide/1  "Driver Power Request (W)"
  Gain/1 -> Divide/2  "Pack Voltage (V)"
  Sony VTC6 Equivalent Circuit/1(Cell Voltage (V)) -> Gain/1  "Cell Voltage (V)"
  Divide/1 -> [pack_current], Pack Current (A)/1  "Pack Current (A)"

== system cbuildv3p1/Battery Thermal Model/Battery Cells/Battery Heat Generation/Pack SoC ==
  Pack Current (A) : Inport
  Constant : Constant  Value=SoC_initial
  Constant1 : Constant  Value=P
  Divide : Product  Inputs=*/
  Gain : Gain  Gain=1/3600
  Integrator : Integrator
  Multiply : Gain  Gain=C_nominal
  Subtract : Sum  Inputs=+-
  SoC (%) : Outport
  tag scope: pack_SOC=global
  wires:
  Pack Current (A)/1 -> Integrator/1
  Constant/1 -> Subtract/1
  Integrator/1 -> Divide/1
  Subtract/1 -> [pack_SOC], SoC (%)/1
  Constant1/1 -> Multiply/1
  Multiply/1 -> Divide/2
  Divide/1 -> Gain/1
  Gain/1 -> Subtract/2

== system cbuildv3p1/Control System/Driver Assists/Torque Vectoring/Target Yaw Rate Estimator ==
  Gain : Gain  Gain=C*2
  Gain1 : Gain  Gain=C*2
  Gain2 : Gain  Gain=a
  Gain3 : Gain  Gain=l-a
  Gain4 : Gain  Gain=-1/Izz
  Slip Angle Estimator : Subsystem
  Sum : Sum  Inputs=|+-
  Yaw Rate Error : Subsystem
      settings: PortSchema="{\"entries\":[{\"content\":{\"sides\":[{\"content\":{},\"type\":\"ConnectorPlacement.EquallySpacedRectSide\",\"uuid\":\"b231141e-075c-44c2-9b61-2a7f1987e8f9\"},{\"content\":{\"side\":\"RIGHT\"},\"type\":\"ConnectorPlacement.EquallySpacedRectSide\",\"uuid\":\"a3423ff2-a1bd-4263-8320-fe535760aa80\"},{\"content\":{\"connectorIds\":[\"In1\"],\"side\":\"TOP\"},\"type\":\"ConnectorPlacement.EquallySpacedRectSide\",\"uuid\":\"1adafbb7-f7c4-42e4-8eab-5e40445049e0\"}]},\"type\":\"ConnectorPlacement.EquallySpacedConnector\",\"uuid\":\"61c95f4c-4142-4f56-9fe1-ea528e3e26a5\"}],\"packageUris\":[\"http://schema.mathworks.com/mf0/Connector/R2020b\"],\"version\":\"1.0\"}"
  tag scope: r_est=global
  wires:
  Gain1/1 -> Gain3/1  "Rear Wheel Lateral Force (N)"
  [alpha_F] -> Gain/1  "Front Wheel Slip Angle (deg)"
  Gain4/1 -> [r_est], Yaw Rate Error/1(r_est)  "Target Yaw Rate (deg/s)"
  Sum/1 -> Gain4/1  "Vehicle Yaw Moment (Nm)"
  Gain2/1 -> Sum/1  "Front Yaw Moment (Nm)"
  Gain/1 -> Gain2/1  "Front Wheel Lateral Force (N)"
  Gain3/1 -> Sum/2  "Rear Yaw Moment (Nm)"
  [alpha_R] -> Gain1/1  "Rear Wheel Slip Angle (deg)"

== system cbuildv3p1/Control System/Driver Assists/Torque Vectoring/Throttle Pedal ==
  P_T : Inport
  Tmax : Inport  Port=2
  Product : Product
  CMD_T : Outport
  wires:
  P_T/1 -> Product/2  "Throttle Pedal Position (-)"
  Product/1 -> CMD_T/1  "Throttle Pedal Torque Command (Nm)"
  Tmax/1 -> Product/1  "Maximum Motor Torque (Nm)"

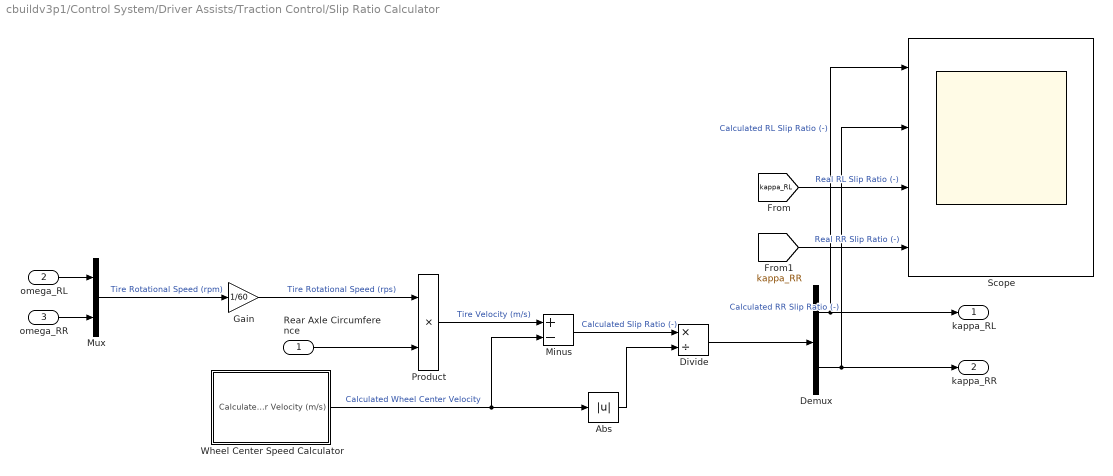
== system cbuildv3p1/Control System/Driver Assists/Traction Control/Slip Ratio Calculator ==
  Rear Axle Circumference : Inport
  omega_RL : Inport  Port=2
  omega_RR : Inport  Port=3
  Abs : Abs  SaturateOnIntegerOverflow=off
  Demux : Demux  Outputs=2
  Divide : Product  Inputs=*/
  Gain : Gain  Gain=1/60
  Minus : Sum  Inputs=+-
  Mux : Mux  Inputs=2
  Product : Product
  Scope : Scope  NumInputPorts=4
  Wheel Center Speed Calculator : Subsystem
  kappa_RL : Outport
  kappa_RR : Outport  Port=2
  wires:
  omega_RL/1 -> Mux/1
  omega_RR/1 -> Mux/2
  Mux/1 -> Gain/1  "Tire Rotational Speed (rpm)"
  Gain/1 -> Product/1  "Tire Rotational Speed (rps)"
  Demux/1 -> kappa_RL/1, Scope/1  "Calculated RL Slip Ratio (-)"
  Demux/2 -> kappa_RR/1, Scope/2  "Calculated RR Slip Ratio (-)"
  [kappa_RL] -> Scope/3  "Real RL Slip Ratio (-)"
  [kappa_RR] -> Scope/4  "Real RR Slip Ratio (-)"
  Product/1 -> Minus/1  "Tire Velocity (m/s)"
  Minus/1 -> Divide/1  "Calculated Slip Ratio (-)"
  Divide/1 -> Demux/1
  Abs/1 -> Divide/2
  Wheel Center Speed Calculator/1(Calculated Wheel Center Velocity (m/s)) -> Minus/2, Abs/1  "Calculated Wheel Center Velocity"
  Rear Axle Circumference/1 -> Product/2

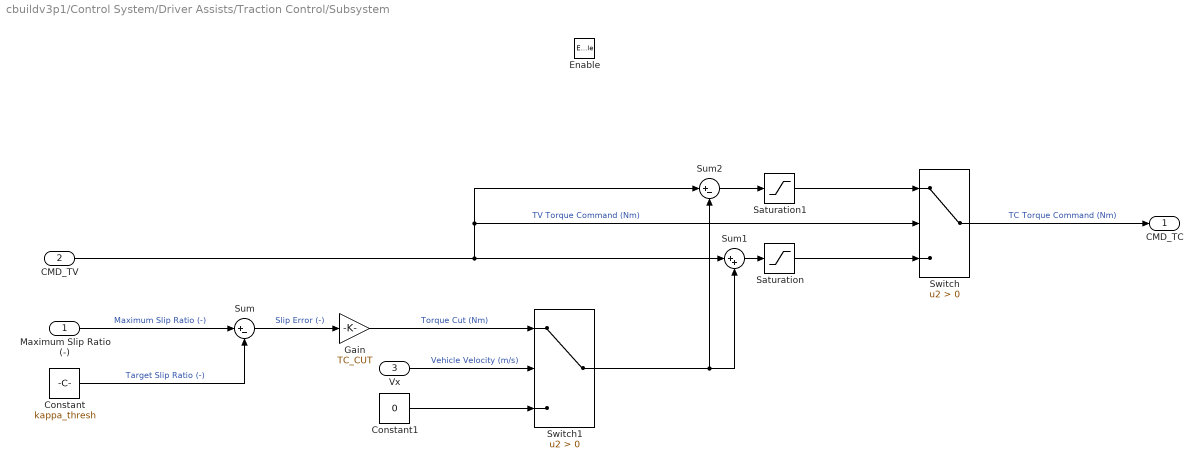
== system cbuildv3p1/Control System/Driver Assists/Traction Control/Subsystem ==
  Maximum Slip Ratio (-) : Inport
  CMD_TV : Inport  Port=2
  Vx : Inport  Port=3
  Enable : EnablePort
  Constant : Constant  Value=kappa_thresh
  Constant1 : Constant  Value=0
  Gain : Gain  Gain=TC_CUT
  Saturation : Saturate  UpperLimit=0  LowerLimit=-Tmax
  Saturation1 : Saturate  UpperLimit=Tmax  LowerLimit=0
  Sum : Sum  Inputs=|+-
  Sum1 : Sum  Inputs=|++
  Sum2 : Sum  Inputs=|+-
  Switch : Switch  Criteria=u2 > Threshold  SaturateOnIntegerOverflow=off  InputSameDT=off
  Switch1 : Switch  Criteria=u2 > Threshold  SaturateOnIntegerOverflow=off  InputSameDT=off
  CMD_TC : Outport
  wires:
  Switch/1 -> CMD_TC/1  "TC Torque Command (Nm)"
  Maximum Slip Ratio (-)/1 -> Sum/1  "Maximum Slip Ratio (-)"
  Constant/1 -> Sum/2  "Target Slip Ratio (-)"
  Sum/1 -> Gain/1  "Slip Error (-)"
  CMD_TV/1 -> Sum2/1, Switch/2, Sum1/1  "TV Torque Command (Nm)"
  Vx/1 -> Switch1/2  "Vehicle Velocity (m/s)"
  Gain/1 -> Switch1/1  "Torque Cut (Nm)"
  Constant1/1 -> Switch1/3
  Switch1/1 -> Sum2/2, Sum1/2
  Sum1/1 -> Saturation/1
  Sum2/1 -> Saturation1/1
  Saturation/1 -> Switch/3
  Saturation1/1 -> Switch/1

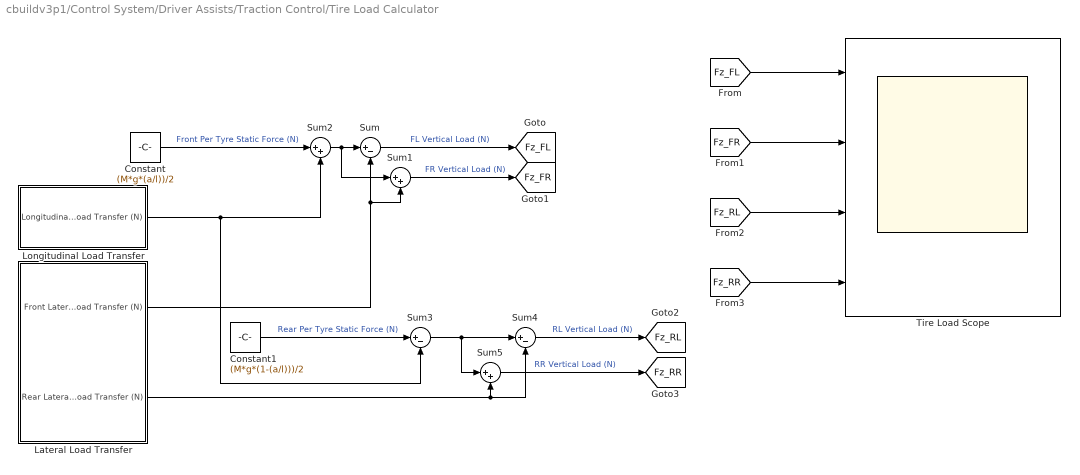
== system cbuildv3p1/Control System/Driver Assists/Traction Control/Tire Load Calculator ==
  Constant : Constant  Value=(M*g*(a/l))/2
  Constant1 : Constant  Value=(M*g*(1-(a/l)))/2
  Lateral Load Transfer : Subsystem
  Longitudinal Load Transfer : Subsystem
  Sum : Sum  Inputs=|+-
  Sum1 : Sum  Inputs=|++
  Sum2 : Sum  Inputs=|++
  Sum3 : Sum  Inputs=|+-
  Sum4 : Sum  Inputs=|+-
  Sum5 : Sum  Inputs=|++
  Tire Load Scope : Scope  NumInputPorts=4
  tag scope: Fz_FL=global, Fz_FR=global, Fz_RL=global, Fz_RR=global
  wires:
  Longitudinal Load Transfer/1(Longitudinal Load Transfer (N)) -> Sum2/2, Sum3/2
  Constant/1 -> Sum2/1  "Front Per Tyre Static Force (N)"
  Sum2/1 -> Sum1/1, Sum/1
  Lateral Load Transfer/1(Front Lateral Load Transfer (N)) -> Sum1/2, Sum/2
  Sum/1 -> [Fz_FL]  "FL Vertical Load (N)"
  Sum1/1 -> [Fz_FR]  "FR Vertical Load (N)"
  Constant1/1 -> Sum3/1  "Rear Per Tyre Static Force (N)"
  Sum3/1 -> Sum5/1, Sum4/1
  Lateral Load Transfer/2(Rear Lateral Load Transfer (N)) -> Sum4/2, Sum5/2
  Sum4/1 -> [Fz_RL]  "RL Vertical Load (N)"
  Sum5/1 -> [Fz_RR]  "RR Vertical Load (N)"
  [Fz_FL] -> Tire Load Scope/1
  [Fz_FR] -> Tire Load Scope/2
  [Fz_RL] -> Tire Load Scope/3
  [Fz_RR] -> Tire Load Scope/4

== system cbuildv3p1/Control System/Driver Assists/Traction Control/Tire Radius Calculator ==
  Constant : Constant  Value=201.094*10^-3
  Constant1 : Constant  Value=2*pi
  Demux : Demux
  Mux : Mux
  Mux1 : Mux  Inputs=2
  Mux2 : Mux  Inputs=2
  Product1 : Product
  Sum : Sum  Inputs=|++
  Tire Stiffness : Gain  Gain=-0.005509*10^-3
  Front Axle Circumference : Outport
  Rear Axle Circumference : Outport  Port=2
  wires:
  Constant1/1 -> Product1/1
  Tire Stiffness/1 -> Sum/1
  Sum/1 -> Product1/2
  Constant/1 -> Sum/2  "Unloaded Tire Radius (m)"
  Mux/1 -> Tire Stiffness/1
  [Fz_FL] -> Mux/1
  [Fz_FR] -> Mux/2
  Product1/1 -> Demux/1  "Tire Circumference (m)"
  [Fz_RL] -> Mux/3
  [Fz_RR] -> Mux/4
  Demux/1 -> Mux1/1
  Demux/4 -> Mux2/2
  Demux/3 -> Mux2/1
  Demux/2 -> Mux1/2
  Mux1/1 -> Front Axle Circumference/1
  Mux2/1 -> Rear Axle Circumference/1

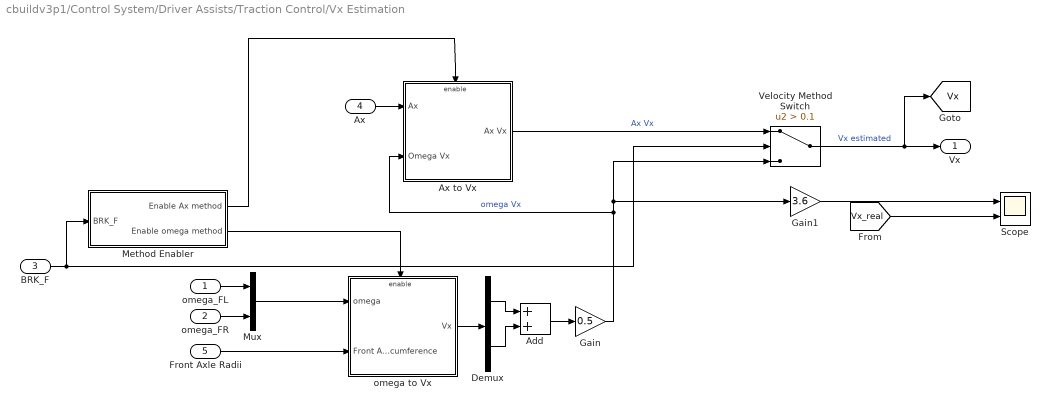
== system cbuildv3p1/Control System/Driver Assists/Traction Control/Vx Estimation ==
  omega_FL : Inport
  omega_FR : Inport  Port=2
  BRK_F : Inport  Port=3
  Ax : Inport  Port=4
  "Front Axle Radii " : Inport  Port=5
  Add : Sum
  Ax to Vx : Subsystem
  Demux : Demux  Outputs=2
  Gain : Gain  Gain=0.5
  Gain1 : Gain  Gain=3.6
  Method Enabler : Subsystem
  Mux : Mux  Inputs=2
  Scope : Scope  NumInputPorts=2
  Velocity Method Switch : Switch  Criteria=u2 > Threshold  Threshold=0.1  SaturateOnIntegerOverflow=off  InputSameDT=off
  omega to Vx : Subsystem
  Vx : Outport
  tag scope: Vx=global
  wires:
  Mux/1 -> omega to Vx/1(omega)
  omega to Vx/1(Vx) -> Demux/1
  Demux/2 -> Add/2
  omega_FR/1 -> Mux/2
  omega_FL/1 -> Mux/1
  Demux/1 -> Add/1
  BRK_F/1 -> Velocity Method Switch/2, Method Enabler/1(BRK_F)
  Add/1 -> Gain/1
  Gain/1 -> Gain1/1, Velocity Method Switch/3, Ax to Vx/2(Omega Vx)  "omega Vx"
  Velocity Method Switch/1 -> [Vx], Vx/1  "Vx estimated"
  Ax/1 -> Ax to Vx/1(Ax)
  Ax to Vx/1(Ax Vx) -> Velocity Method Switch/1  "Ax Vx"
  Method Enabler/2(Enable omega method) -> omega to Vx/Enable
  Method Enabler/1(Enable Ax method) -> Ax to Vx/Enable
  "Front Axle Radii "/1 -> omega to Vx/2(Front Axle Circumference)
  [Vx_real] -> Scope/2
  Gain1/1 -> Scope/1

== system cbuildv3p1/Control System/Energy Management System/Dynamic Derate/Motor Torque Calculator ==
  omega_RL : Inport
  omega_RR : Inport  Port=2
  B_MAX : Inport  Port=3
  Add : Sum
  Divide : Product  Inputs=*/
  Gain : Gain  Gain=0.5
  Gain1 : Gain  Gain=pi/30
  Gain2 : Gain  Gain=500
  Gain3 : Gain  Gain=GR
  Tmax : Outport
  wires:
  omega_RR/1 -> Add/2  "RR Wheel Speed (rpm)"
  Add/1 -> Gain/1
  omega_RL/1 -> Add/1  "RL Wheel Speed (rpm)"
  Gain/1 -> Gain3/1
  Gain1/1 -> Divide/2
  B_MAX/1 -> Gain2/1  "Maximum Battery Power (KW)"
  Divide/1 -> Tmax/1
  Gain2/1 -> Divide/1
  Gain3/1 -> Gain1/1

== system cbuildv3p1/Battery Thermal Model/Battery Cells/Battery Heat Generation/Pack Current/Power Estimator ==
  Abs : Abs  SaturateOnIntegerOverflow=off
  Abs1 : Abs  SaturateOnIntegerOverflow=off
  Add : Sum
  Gain : Gain  Gain=rpm_to_radpers * GR
  Gain2 : Gain  Gain=rpm_to_radpers * GR
  Product : Product
  Product1 : Product
  Motor Power (W) : Outport
  wires:
  [omega_RL] -> Gain/1
  [CMD_RL] -> Product/1
  Gain/1 -> Product/2
  Gain2/1 -> Product1/2
  [CMD_RR] -> Product1/1
  [omega_RR] -> Gain2/1
  Product/1 -> Abs/1  "Left Motor Power (W)"
  Product1/1 -> Abs1/1  "Right Motor Power (W)"
  Add/1 -> Motor Power (W)/1  "Motor Power (W)"
  Abs/1 -> Add/1
  Abs1/1 -> Add/2

== system cbuildv3p1/Battery Thermal Model/Battery Cells/Battery Heat Generation/Pack Current/Sony VTC6 Equivalent Circuit ==
  Divide : Product  Inputs=*/
  Equivalent Circuit Look Ups : Subsystem
  Gain : Gain  Gain=1/(P * C_nominal)
  Gain1 : Gain  Gain=1/(P*S)
  Product : Product
  Subtract : Sum  Inputs=+-
  fitment gain : Gain  Gain=sqrt(5)
  Cell Voltage (V) : Outport
  tag scope: OCV=global, cell_voltage=global
  wires:
  [pack_SOC] -> Equivalent Circuit Look Ups/1(Pack SoC (-))  "Pack SoC (-)"
  Gain/1 -> Equivalent Circuit Look Ups/2(Cell C-Rate (-))  "Cell C-Rate (-)"
  Equivalent Circuit Look Ups/2(R0 Resistance (ohms)) -> fitment gain/1  "R0 Resistance (Ohms)"
  Equivalent Circuit Look Ups/1(OCV (V)) -> [OCV], Subtract/1, Divide/2  "Open Circuit Voltage (V)"
  Product/1 -> Subtract/2  "R0 Voltage Loss (V)"
  Subtract/1 -> [cell_voltage], Cell Voltage (V)/1  "Cell Voltage (V)"
  Divide/1 -> Product/2  "Initial Current Guess (A)"
  [power_lol] -> Gain1/1  "Pack Power Request (W)"
  Gain1/1 -> Divide/1  "Cell Power Request (W)"
  [pack_current] -> Gain/1  "Pack Current (A)"
  fitment gain/1 -> Product/1

== system cbuildv3p1/Control System/Driver Assists/Torque Vectoring/Target Yaw Rate Estimator/Slip Angle Estimator ==
  note: \arctan\left(\frac{a}{R}\right)
  Front : Subsystem
  Rear : Subsystem

== system cbuildv3p1/Control System/Driver Assists/Torque Vectoring/Target Yaw Rate Estimator/Yaw Rate Error ==
  r_est : Inport
  Mux : Mux  Inputs=2
  Sum : Sum  Inputs=|+-
  Yaw Rate Scope : Scope
  tag scope: r_error=global
  wires:
  r_est/1 -> Mux/1, Sum/1  "Target Yaw Rate (deg/s)"
  [r] -> Mux/2, Sum/2  "Yaw Rate (deg/s)"
  Sum/1 -> [r_error]  "Yaw Rate Error (deg/s)"
  Mux/1 -> Yaw Rate Scope/1

== system cbuildv3p1/Control System/Driver Assists/Traction Control/Slip Ratio Calculator/Wheel Center Speed Calculator ==
  Gain : Gain  Gain=t/2
  Gain1 : Gain  Gain=deg_to_rad
  Mux : Mux  Inputs=2
  Sum : Sum  Inputs=|++
  Sum1 : Sum  Inputs=|+-
  Calculated Wheel Center Velocity (m/s) : Outport
  wires:
  [r] -> Gain1/1  "Yaw Rate (deg/s)"
  [Vx] -> Sum1/1, Sum/2  "Vehicle Velocity (m/s)"
  Mux/1 -> Calculated Wheel Center Velocity (m/s)/1
  Gain/1 -> Sum/1, Sum1/2
  Sum1/1 -> Mux/1  "RL WC Velocity (m/s)"
  Gain1/1 -> Gain/1  "Yaw Rate (rad/s)"
  Sum/1 -> Mux/2  "RR WC Velocity (m/s)"

== system cbuildv3p1/Control System/Driver Assists/Traction Control/Tire Load Calculator/Lateral Load Transfer ==
  Constant : Constant  Value=h
  Constant1 : Constant  Value=t
  Divide : Product  Inputs=*/
  Gain1 : Gain  Gain=M*g*(a/l)
  Gain2 : Gain  Gain=M*g*(1- (a/l))
  Product : Product
  Front Lateral Load Transfer (N) : Outport
  Rear Lateral Load Transfer (N) : Outport  Port=2
  wires:
  [Ay] -> Product/1  "Lateral Acceleration (G)"
  Constant/1 -> Product/2  "CG Height (m)"
  Product/1 -> Divide/1
  Constant1/1 -> Divide/2  "Trackwidth (m)"
  Gain1/1 -> Front Lateral Load Transfer (N)/1  "Front Lateral Load Transfer (N)"
  Divide/1 -> Gain2/1, Gain1/1
  Gain2/1 -> Rear Lateral Load Transfer (N)/1  "Rear Lateral Load Transfer (N)"

== system cbuildv3p1/Control System/Driver Assists/Traction Control/Tire Load Calculator/Longitudinal Load Transfer ==
  Gain : Gain  Gain=-h/W
  Gain1 : Gain  Gain=M*g
  Longitudinal Load Transfer (N) : Outport
  wires:
  [Ax] -> Gain/1
  Gain/1 -> Gain1/1
  Gain1/1 -> Longitudinal Load Transfer (N)/1

== system cbuildv3p1/Control System/Driver Assists/Traction Control/Vx Estimation/Ax to Vx ==
  Ax : Inport
  Omega Vx : Inport  Port=2
  Enable : EnablePort
  Integrator : Integrator
  Plus : Sum
  to m/s^2 : Gain  Gain=g
  Ax Vx : Outport
  wires:
  Ax/1 -> to m/s^2/1
  Integrator/1 -> Plus/2
  Omega Vx/1 -> Plus/1
  Plus/1 -> Ax Vx/1
  to m/s^2/1 -> Integrator/1
